simulink model "IEEE33BusTestSystem_DG_Ident"  (R2019a)
settings: Solver=VariableStepAuto  StartTime=0.0  StopTime=1.5  FixedStep=5e-5  RelTol=1e-3
values from neighbouring files (symbols this model uses):
  P_dg0 = 300*ones(1,6)    [IEEE33BusSystem_Control_Sim.m]    (also in IEEE33BusSystem_Control_Sim_nq3.m; IEEE33BusSystem_Control_Sim_nq5.m; IEEE33BusSystem_Ident.m; IEEE33BusSystem_op.m)
  P_dgf = 100*ones(1,6)    [IEEE33BusSystem_Control_Sim.m]    (also in IEEE33BusSystem_Control_Sim_nq3.m; IEEE33BusSystem_Control_Sim_nq5.m; IEEE33BusSystem_op.m = 300*ones(1,6); Kimc_d1_sce1-0.mat = [100 100 100 100 100 100])
  Q_dg0 = zeros(1,6)    [IEEE33BusSystem_Control_Sim.m]    (also in IEEE33BusSystem_Control_Sim_nq3.m; IEEE33BusSystem_Control_Sim_nq5.m; IEEE33BusSystem_Ident.m; IEEE33BusSystem_op.m)
  Q_dgf = zeros(1,6)    [IEEE33BusSystem_op.m]
  Tp = 500e-3    (= 0.5)    [IEEE33BusSystem.m]    (also in Kimc_d1_sce1-0.mat = 0.05; Kimc_d1_sce1-1.mat = 0.05; Kimc_d1_sce1-2.mat = 0.05; Kimc_d1_sce1-3.mat = 0.05)
  tPdg = 10*ones(1,6)    [IEEE33BusSystem_Control_Sim.m]    (also in IEEE33BusSystem_Control_Sim_nq3.m; IEEE33BusSystem_Control_Sim_nq5.m; IEEE33BusSystem_op.m = 0.5*ones(1,6); Kimc_d1_sce1-0.mat = [10 10 10 10 10 10])
  Tq = 50e-3    (= 0.05)    [IEEE33BusSystem.m]    (also in Kimc_d1_sce1-0.mat; Kimc_d1_sce1-1.mat; Kimc_d1_sce1-2.mat; Kimc_d1_sce1-3.mat)
  tQdg = 0.5*ones(1,6)    [IEEE33BusSystem_op.m]
  v0 = ones(1,33)    [IEEE33BusSystem_Control_Sim.m]    (also in IEEE33BusSystem_Control_Sim_nq3.m; IEEE33BusSystem_Control_Sim_nq5.m; IEEE33BusSystem_Ident.m; IEEE33BusSystem_op.m)
  V_0 = v0_sim(CVs_sel)    [IEEE33BusSystem_Control_Sim.m]    (also in IEEE33BusSystem_Control_Sim_nq3.m = [v0_sim(14), v0_sim(18), v0_sim(21), v0_sim(25), v0_sim(30),; IEEE33BusSystem_Control_Sim_nq5.m = [v0_sim(14), v0_sim(18), v0_sim(21), v0_sim(25), v0_sim(30),; IEEE33BusSystem_Ident.m; IEEE33BusSystem_op.m = [v0(14), v0(18), v0(21), v0(25), v0(30), v0(33)])
libraries: powerlib x159, powerlib_meascontrol x33
(part 3 of 3)

== system IEEE33BusTestSystem_DG_Ident/Bus_32 ==
  Bus Load 32 : powerlib/Elements/Three-Phase Series RLC Load  LConnTagsString=A|B|C  Configuration=Y (grounded)  NominalVoltage=(12660)*v0(32)  Vabc=[1e3 1e3 1e3]  Vabcp=[1e3 1e3 1e3]  NominalFrequency=50  UnbalancedPower=off  ActivePower=210e3  InductivePower=100e3  CapacitivePower=0  Pabc=[10e3 9e3 11e3]  QLabc=[100 90 110]  QCabc=[100 90 110]  Pabcp=[10e3 9e3 11e3]  QLabcp=[100 90 110]  QCabcp=[100 90 110]  Measurements=None  LoadType=constant PQ
      settings: SourceProductName=Simscape Electrical
  Bus_32 : powerlib/Measurements/Three-Phase V-I Measurement  VoltageMeasurement=phase-to-phase  SetLabelV=on  LabelV=v32_pu  Vpu=off  VpuLL=on  CurrentMeasurement=yes  SetLabelI=on  LabelI=I3132_pu  Ipu=off  Pbase=100e6  Vbase=12660  OutputType=Complex  PhasorSimulation=on  PSBequivalent=0
      settings: SourceProductName=Simscape Electrical
  CB3-2 : powerlib/Elements/Three-Phase Breaker  InitialState=open  SwitchA=on  SwitchB=on  SwitchC=on  SwitchTimes="[1/60  5/60]"  External=on  BreakerResistance=0.01  SnubberResistance=1e6  SnubberCapacitance=inf  Measurements=None
      settings: SourceProductName=Simscape Electrical
  InPhaseA : PMIOPort  Side=Left
  InPhaseB : PMIOPort  Port=2  Side=Left
  InPhaseC : PMIOPort  Port=3  Side=Left
  OutPhaseA : PMIOPort  Port=4  Side=Right
  OutPhaseB : PMIOPort  Port=5  Side=Right
  OutPhaseC : PMIOPort  Port=6  Side=Right
  wires:
  [CB32to33] -> CB3-2/1
  connections:
  Bus_32/RConn1 -- CB3-2/LConn1 -- Bus Load 32/LConn1
  CB3-2/RConn3 -- OutPhaseC/RConn1
  Bus Load 32/LConn2 -- CB3-2/LConn2 -- Bus_32/RConn2
  Bus_32/RConn3 -- Bus Load 32/LConn3 -- CB3-2/LConn3
  CB3-2/RConn1 -- OutPhaseA/RConn1
  CB3-2/RConn2 -- OutPhaseB/RConn1
  InPhaseA/RConn1 -- Bus_32/LConn1
  InPhaseB/RConn1 -- Bus_32/LConn2
  InPhaseC/RConn1 -- Bus_32/LConn3

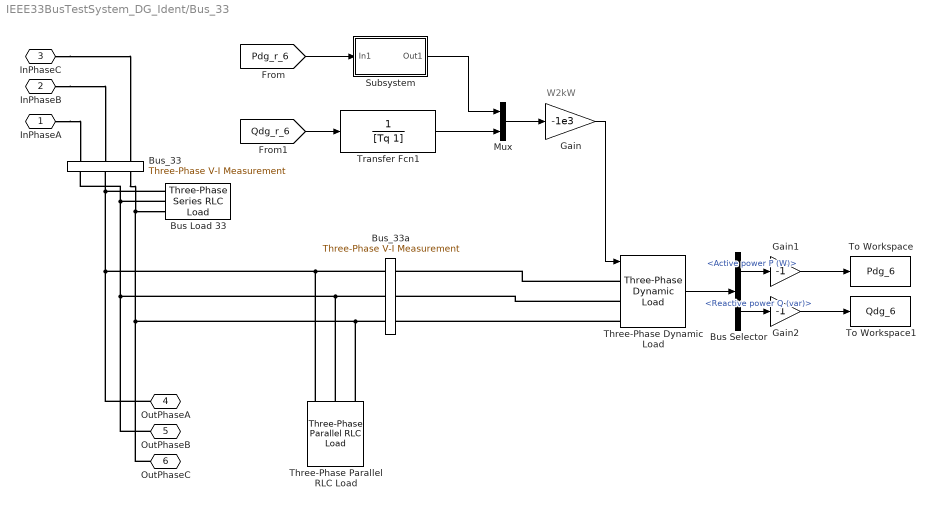
== system IEEE33BusTestSystem_DG_Ident/Bus_33 ==
  note: W2kW
  Bus Load 33 : powerlib/Elements/Three-Phase Series RLC Load  LConnTagsString=A|B|C  Configuration=Y (grounded)  NominalVoltage=(12660)*v0(33)  Vabc=[1e3 1e3 1e3]  Vabcp=[1e3 1e3 1e3]  NominalFrequency=50  UnbalancedPower=off  ActivePower=60e3  InductivePower=40e3  CapacitivePower=0  Pabc=[10e3 9e3 11e3]  QLabc=[100 90 110]  QCabc=[100 90 110]  Pabcp=[10e3 9e3 11e3]  QLabcp=[100 90 110]  QCabcp=[100 90 110]  Measurements=None  LoadType=constant PQ
      settings: SourceProductName=Simscape Electrical
  Bus Selector : BusSelector  OutputSignals=Active power P (W),Reactive power Q (var)
  Bus_33 : powerlib/Measurements/Three-Phase V-I Measurement  VoltageMeasurement=phase-to-phase  SetLabelV=on  LabelV=v33_pu  Vpu=off  VpuLL=on  CurrentMeasurement=yes  SetLabelI=on  LabelI=Iabc  Ipu=off  Pbase=100e6  Vbase=12660  OutputType=Complex  PhasorSimulation=on  PSBequivalent=0
      settings: SourceProductName=Simscape Electrical
  Bus_33a : powerlib/Measurements/Three-Phase V-I Measurement  VoltageMeasurement=no  SetLabelV=off  LabelV=v14a_pu  Vpu=off  VpuLL=off  CurrentMeasurement=yes  SetLabelI=on  LabelI=I33a_pu  Ipu=off  Pbase=100e6  Vbase=500e3  OutputType=Complex  PhasorSimulation=on  PSBequivalent=0
      settings: SourceProductName=Simscape Electrical
  Gain : Gain  Gain=-1e3
  Gain1 : Gain  Gain=-1
  Gain2 : Gain  Gain=-1
  Mux : Mux  Inputs=2
  Subsystem : Subsystem
  Three-Phase Dynamic Load : powerlib/Elements/Three-Phase Dynamic Load  NominalVoltage=[ 12660 50 ]  ActiveReactivePowers=[-P_dg0(6) Q_dg0(6)]*1e3  PositiveSequence=[V_0(6) 0]  ExternalControl=on  NpNq=[1.3 2]  TimeConstants="[0  0  0  0]"  MinimumVoltage=0.7  Tfilter=1e-4  LoadFlowParameters=[4,0,0,0,0]
      settings: SourceProductName=Simscape Electrical  SourceProductBaseCode=PS
  Three-Phase Parallel RLC Load : powerlib/Elements/Three-Phase Parallel RLC Load  LConnTagsString=A|B|C  Configuration=Y (grounded)  NominalVoltage=12660  Vabc=[1e3 1e3 1e3]  Vabcp=[1e3 1e3 1e3]  NominalFrequency=50  UnbalancedPower=off  ActivePower=0.01  InductivePower=0  CapacitivePower=0  Pabc=[10e3 9e3 11e3]  QLabc=[100 90 110]  QCabc=[100 90 110]  Pabcp=[10e3 9e3 11e3]  QLabcp=[100 90 110]  QCabcp=[100 90 110]  Measurements=None  LoadType=constant Z
      settings: SourceProductName=Simscape Electrical
  To Workspace : ToWorkspace  VariableName=Pdg_6  SaveFormat=Timeseries  SampleTime=-1
  To Workspace1 : ToWorkspace  VariableName=Qdg_6  SaveFormat=Timeseries  SampleTime=-1
  Transfer Fcn1 : TransferFcn  Denominator=[Tq 1]
  InPhaseA : PMIOPort  Side=Left
  InPhaseB : PMIOPort  Port=2  Side=Left
  InPhaseC : PMIOPort  Port=3  Side=Left
  OutPhaseA : PMIOPort  Port=4  Side=Right
  OutPhaseB : PMIOPort  Port=5  Side=Right
  OutPhaseC : PMIOPort  Port=6  Side=Right
  wires:
  Subsystem/1(Out1) -> Mux/1
  Transfer Fcn1/1 -> Mux/2
  Bus Selector/1 -> Gain1/1  "<Active power P (W)>"
  [Pdg_r_6] -> Subsystem/1(In1)
  Gain2/1 -> To Workspace1/1
  Bus Selector/2 -> Gain2/1  "<Reactive power Q (var)>"
  Mux/1 -> Gain/1
  Three-Phase Dynamic Load/1 -> Bus Selector/1
  Gain/1 -> Three-Phase Dynamic Load/1
  Gain1/1 -> To Workspace/1
  [Qdg_r_6] -> Transfer Fcn1/1
  connections:
  Bus Load 33/LConn1 -- Three-Phase Parallel RLC Load/LConn1 -- Bus_33a/RConn1 -- OutPhaseA/RConn1 -- Bus_33/RConn1
  Bus Load 33/LConn2 -- Three-Phase Parallel RLC Load/LConn2 -- Bus_33a/RConn2 -- OutPhaseB/RConn1 -- Bus_33/RConn2
  Bus_33/RConn3 -- Three-Phase Parallel RLC Load/LConn3 -- Bus_33a/RConn3 -- OutPhaseC/RConn1 -- Bus Load 33/LConn3
  InPhaseA/RConn1 -- Bus_33/LConn1
  InPhaseB/RConn1 -- Bus_33/LConn2
  InPhaseC/RConn1 -- Bus_33/LConn3
  Three-Phase Dynamic Load/LConn1 -- Bus_33a/LConn1
  Three-Phase Dynamic Load/LConn3 -- Bus_33a/LConn3
  Three-Phase Dynamic Load/LConn2 -- Bus_33a/LConn2

== system IEEE33BusTestSystem_DG_Ident/Bus_4 ==
  Bus Load 4 : powerlib/Elements/Three-Phase Series RLC Load  LConnTagsString=A|B|C  Configuration=Y (grounded)  NominalVoltage=(12660)*v0(4)  Vabc=[1e3 1e3 1e3]  Vabcp=[1e3 1e3 1e3]  NominalFrequency=50  UnbalancedPower=off  ActivePower=120e3  InductivePower=80e3  CapacitivePower=0  Pabc=[10e3 9e3 11e3]  QLabc=[100 90 110]  QCabc=[100 90 110]  Pabcp=[10e3 9e3 11e3]  QLabcp=[100 90 110]  QCabcp=[100 90 110]  Measurements=None  LoadType=constant PQ
      settings: SourceProductName=Simscape Electrical
  Bus_4 : powerlib/Measurements/Three-Phase V-I Measurement  VoltageMeasurement=phase-to-phase  SetLabelV=on  LabelV=v4_pu  Vpu=off  VpuLL=on  CurrentMeasurement=yes  SetLabelI=on  LabelI=I34_pu  Ipu=off  Pbase=10e6  Vbase=12660  OutputType=Complex  PhasorSimulation=on  PSBequivalent=0
      settings: SourceProductName=Simscape Electrical
  CB3-2 : powerlib/Elements/Three-Phase Breaker  InitialState=open  SwitchA=on  SwitchB=on  SwitchC=on  SwitchTimes="[1/60  5/60]"  External=on  BreakerResistance=0.01  SnubberResistance=1e6  SnubberCapacitance=inf  Measurements=None
      settings: SourceProductName=Simscape Electrical
  InPhaseA : PMIOPort  Side=Left
  InPhaseB : PMIOPort  Port=2  Side=Left
  InPhaseC : PMIOPort  Port=3  Side=Left
  OutPhaseA : PMIOPort  Port=4  Side=Right
  OutPhaseB : PMIOPort  Port=5  Side=Right
  OutPhaseC : PMIOPort  Port=6  Side=Right
  wires:
  [CB4to5] -> CB3-2/1
  connections:
  Bus_4/RConn1 -- CB3-2/LConn1 -- Bus Load 4/LConn1
  CB3-2/RConn3 -- OutPhaseC/RConn1
  Bus Load 4/LConn2 -- CB3-2/LConn2 -- Bus_4/RConn2
  Bus_4/RConn3 -- CB3-2/LConn3 -- Bus Load 4/LConn3
  CB3-2/RConn1 -- OutPhaseA/RConn1
  CB3-2/RConn2 -- OutPhaseB/RConn1
  InPhaseA/RConn1 -- Bus_4/LConn1
  InPhaseB/RConn1 -- Bus_4/LConn2
  InPhaseC/RConn1 -- Bus_4/LConn3

== system IEEE33BusTestSystem_DG_Ident/Bus_5 ==
  Bus Load 5 : powerlib/Elements/Three-Phase Series RLC Load  LConnTagsString=A|B|C  Configuration=Y (grounded)  NominalVoltage=(12660)*v0(5)  Vabc=[1e3 1e3 1e3]  Vabcp=[1e3 1e3 1e3]  NominalFrequency=50  UnbalancedPower=off  ActivePower=60e3  InductivePower=30e3  CapacitivePower=0  Pabc=[10e3 9e3 11e3]  QLabc=[100 90 110]  QCabc=[100 90 110]  Pabcp=[10e3 9e3 11e3]  QLabcp=[100 90 110]  QCabcp=[100 90 110]  Measurements=None  LoadType=constant PQ
      settings: SourceProductName=Simscape Electrical
  Bus_5 : powerlib/Measurements/Three-Phase V-I Measurement  VoltageMeasurement=phase-to-phase  SetLabelV=on  LabelV=v5_pu  Vpu=off  VpuLL=on  CurrentMeasurement=yes  SetLabelI=on  LabelI=I45_pu  Ipu=off  Pbase=10e6  Vbase=12660  OutputType=Complex  PhasorSimulation=on  PSBequivalent=0
      settings: SourceProductName=Simscape Electrical
  CB3-2 : powerlib/Elements/Three-Phase Breaker  InitialState=open  SwitchA=on  SwitchB=on  SwitchC=on  SwitchTimes="[1/60  5/60]"  External=on  BreakerResistance=0.01  SnubberResistance=1e6  SnubberCapacitance=inf  Measurements=None
      settings: SourceProductName=Simscape Electrical
  InPhaseA : PMIOPort  Side=Left
  InPhaseB : PMIOPort  Port=2  Side=Left
  InPhaseC : PMIOPort  Port=3  Side=Left
  OutPhaseA : PMIOPort  Port=4  Side=Right
  OutPhaseB : PMIOPort  Port=5  Side=Right
  OutPhaseC : PMIOPort  Port=6  Side=Right
  wires:
  [CB5to6] -> CB3-2/1
  connections:
  Bus Load 5/LConn1 -- CB3-2/LConn1 -- Bus_5/RConn1
  CB3-2/RConn3 -- OutPhaseC/RConn1
  Bus_5/RConn2 -- CB3-2/LConn2 -- Bus Load 5/LConn2
  Bus_5/RConn3 -- CB3-2/LConn3 -- Bus Load 5/LConn3
  CB3-2/RConn1 -- OutPhaseA/RConn1
  CB3-2/RConn2 -- OutPhaseB/RConn1
  InPhaseA/RConn1 -- Bus_5/LConn1
  InPhaseB/RConn1 -- Bus_5/LConn2
  InPhaseC/RConn1 -- Bus_5/LConn3

== system IEEE33BusTestSystem_DG_Ident/Bus_6 ==
  Bus Load 6 : powerlib/Elements/Three-Phase Series RLC Load  LConnTagsString=A|B|C  Configuration=Y (grounded)  NominalVoltage=(12660)*v0(6)  Vabc=[1e3 1e3 1e3]  Vabcp=[1e3 1e3 1e3]  NominalFrequency=50  UnbalancedPower=off  ActivePower=60e3  InductivePower=20e3  CapacitivePower=0  Pabc=[10e3 9e3 11e3]  QLabc=[100 90 110]  QCabc=[100 90 110]  Pabcp=[10e3 9e3 11e3]  QLabcp=[100 90 110]  QCabcp=[100 90 110]  Measurements=None  LoadType=constant PQ
      settings: SourceProductName=Simscape Electrical
  Bus_6 : powerlib/Measurements/Three-Phase V-I Measurement  VoltageMeasurement=phase-to-phase  SetLabelV=on  LabelV=v6_pu  Vpu=off  VpuLL=on  CurrentMeasurement=yes  SetLabelI=on  LabelI=I56_pu  Ipu=off  Pbase=100e6  Vbase=12660  OutputType=Complex  PhasorSimulation=on  PSBequivalent=0
      settings: SourceProductName=Simscape Electrical
  CB3-1 : powerlib/Elements/Three-Phase Breaker  InitialState=open  SwitchA=on  SwitchB=on  SwitchC=on  SwitchTimes="[1/60  5/60]"  External=on  BreakerResistance=0.01  SnubberResistance=1e6  SnubberCapacitance=inf  Measurements=None
      settings: SourceProductName=Simscape Electrical
  CB3-2 : powerlib/Elements/Three-Phase Breaker  InitialState=open  SwitchA=on  SwitchB=on  SwitchC=on  SwitchTimes="[1/60  5/60]"  External=on  BreakerResistance=0.01  SnubberResistance=1e6  SnubberCapacitance=inf  Measurements=None
      settings: SourceProductName=Simscape Electrical
  InPhaseA : PMIOPort  Side=Left
  InPhaseB : PMIOPort  Port=2  Side=Left
  InPhaseC : PMIOPort  Port=3  Side=Left
  OutPhaseA : PMIOPort  Port=4  Side=Right
  OutPhaseB : PMIOPort  Port=5  Side=Right
  OutPhaseC : PMIOPort  Port=6  Side=Right
  OutPhaseA1 : PMIOPort  Port=7  Side=Right
  OutPhaseB1 : PMIOPort  Port=8  Side=Right
  OutPhaseC1 : PMIOPort  Port=9  Side=Right
  wires:
  [CB6to26] -> CB3-1/1
  [CB6to7] -> CB3-2/1
  connections:
  Bus Load 6/LConn1 -- Bus_6/RConn1 -- CB3-2/LConn1 -- CB3-1/LConn1
  CB3-2/RConn3 -- OutPhaseC/RConn1
  Bus Load 6/LConn2 -- Bus_6/RConn2 -- CB3-1/LConn2 -- CB3-2/LConn2
  Bus Load 6/LConn3 -- Bus_6/RConn3 -- CB3-1/LConn3 -- CB3-2/LConn3
  CB3-2/RConn1 -- OutPhaseA/RConn1
  CB3-2/RConn2 -- OutPhaseB/RConn1
  CB3-1/RConn3 -- OutPhaseC1/RConn1
  CB3-1/RConn2 -- OutPhaseB1/RConn1
  CB3-1/RConn1 -- OutPhaseA1/RConn1
  InPhaseA/RConn1 -- Bus_6/LConn1
  InPhaseB/RConn1 -- Bus_6/LConn2
  InPhaseC/RConn1 -- Bus_6/LConn3

== system IEEE33BusTestSystem_DG_Ident/Bus_7 ==
  Bus Load 7 : powerlib/Elements/Three-Phase Series RLC Load  LConnTagsString=A|B|C  Configuration=Y (grounded)  NominalVoltage=(12660)*v0(7)  Vabc=[1e3 1e3 1e3]  Vabcp=[1e3 1e3 1e3]  NominalFrequency=50  UnbalancedPower=off  ActivePower=200e3  InductivePower=100e3  CapacitivePower=0  Pabc=[10e3 9e3 11e3]  QLabc=[100 90 110]  QCabc=[100 90 110]  Pabcp=[10e3 9e3 11e3]  QLabcp=[100 90 110]  QCabcp=[100 90 110]  Measurements=None  LoadType=constant PQ
      settings: SourceProductName=Simscape Electrical
  Bus_7 : powerlib/Measurements/Three-Phase V-I Measurement  VoltageMeasurement=phase-to-phase  SetLabelV=on  LabelV=v7_pu  Vpu=off  VpuLL=on  CurrentMeasurement=yes  SetLabelI=on  LabelI=I67_pu  Ipu=off  Pbase=100e6  Vbase=12660  OutputType=Complex  PhasorSimulation=on  PSBequivalent=0
      settings: SourceProductName=Simscape Electrical
  CB3-2 : powerlib/Elements/Three-Phase Breaker  InitialState=open  SwitchA=on  SwitchB=on  SwitchC=on  SwitchTimes="[1/60  5/60]"  External=on  BreakerResistance=0.01  SnubberResistance=1e6  SnubberCapacitance=inf  Measurements=None
      settings: SourceProductName=Simscape Electrical
  InPhaseA : PMIOPort  Side=Left
  InPhaseB : PMIOPort  Port=2  Side=Left
  InPhaseC : PMIOPort  Port=3  Side=Left
  OutPhaseA : PMIOPort  Port=4  Side=Right
  OutPhaseB : PMIOPort  Port=5  Side=Right
  OutPhaseC : PMIOPort  Port=6  Side=Right
  wires:
  [CB7to8] -> CB3-2/1
  connections:
  Bus_7/RConn1 -- CB3-2/LConn1 -- Bus Load 7/LConn1
  CB3-2/RConn3 -- OutPhaseC/RConn1
  Bus Load 7/LConn2 -- CB3-2/LConn2 -- Bus_7/RConn2
  CB3-2/LConn3 -- Bus Load 7/LConn3 -- Bus_7/RConn3
  CB3-2/RConn1 -- OutPhaseA/RConn1
  CB3-2/RConn2 -- OutPhaseB/RConn1
  InPhaseA/RConn1 -- Bus_7/LConn1
  InPhaseB/RConn1 -- Bus_7/LConn2
  InPhaseC/RConn1 -- Bus_7/LConn3

== system IEEE33BusTestSystem_DG_Ident/Bus_8 ==
  Bus Load 8 : powerlib/Elements/Three-Phase Series RLC Load  LConnTagsString=A|B|C  Configuration=Y (grounded)  NominalVoltage=(12660)*v0(8)  Vabc=[1e3 1e3 1e3]  Vabcp=[1e3 1e3 1e3]  NominalFrequency=50  UnbalancedPower=off  ActivePower=200e3  InductivePower=100e3  CapacitivePower=0  Pabc=[10e3 9e3 11e3]  QLabc=[100 90 110]  QCabc=[100 90 110]  Pabcp=[10e3 9e3 11e3]  QLabcp=[100 90 110]  QCabcp=[100 90 110]  Measurements=None  LoadType=constant PQ
      settings: SourceProductName=Simscape Electrical
  Bus_8 : powerlib/Measurements/Three-Phase V-I Measurement  VoltageMeasurement=phase-to-phase  SetLabelV=on  LabelV=v8_pu  Vpu=off  VpuLL=on  CurrentMeasurement=yes  SetLabelI=on  LabelI=I78_pu  Ipu=off  Pbase=100e6  Vbase=12660  OutputType=Complex  PhasorSimulation=on  PSBequivalent=0
      settings: SourceProductName=Simscape Electrical
  CB3-2 : powerlib/Elements/Three-Phase Breaker  InitialState=open  SwitchA=on  SwitchB=on  SwitchC=on  SwitchTimes="[1/60  5/60]"  External=on  BreakerResistance=0.01  SnubberResistance=1e6  SnubberCapacitance=inf  Measurements=None
      settings: SourceProductName=Simscape Electrical
  InPhaseA : PMIOPort  Side=Left
  InPhaseB : PMIOPort  Port=2  Side=Left
  InPhaseC : PMIOPort  Port=3  Side=Left
  OutPhaseA : PMIOPort  Port=4  Side=Right
  OutPhaseB : PMIOPort  Port=5  Side=Right
  OutPhaseC : PMIOPort  Port=6  Side=Right
  InPhaseA1 : PMIOPort  Port=7  Side=Left
  InPhaseB1 : PMIOPort  Port=8  Side=Left
  InPhaseC1 : PMIOPort  Port=9  Side=Left
  wires:
  [CB8to9] -> CB3-2/1
  connections:
  Bus Load 8/LConn1 -- CB3-2/LConn1 -- Bus_8/RConn1
  CB3-2/RConn3 -- OutPhaseC/RConn1
  Bus Load 8/LConn2 -- CB3-2/LConn2 -- Bus_8/RConn2
  Bus_8/RConn3 -- CB3-2/LConn3 -- Bus Load 8/LConn3
  CB3-2/RConn1 -- OutPhaseA/RConn1
  CB3-2/RConn2 -- OutPhaseB/RConn1
  InPhaseA1/RConn1 -- InPhaseA/RConn1 -- Bus_8/LConn1
  InPhaseB1/RConn1 -- InPhaseB/RConn1 -- Bus_8/LConn2
  InPhaseC1/RConn1 -- InPhaseC/RConn1 -- Bus_8/LConn3

== system IEEE33BusTestSystem_DG_Ident/Bus_9 ==
  Bus Load 9 : powerlib/Elements/Three-Phase Series RLC Load  LConnTagsString=A|B|C  Configuration=Y (grounded)  NominalVoltage=(12660)*v0(9)  Vabc=[1e3 1e3 1e3]  Vabcp=[1e3 1e3 1e3]  NominalFrequency=50  UnbalancedPower=off  ActivePower=60e3  InductivePower=20e3  CapacitivePower=0  Pabc=[10e3 9e3 11e3]  QLabc=[100 90 110]  QCabc=[100 90 110]  Pabcp=[10e3 9e3 11e3]  QLabcp=[100 90 110]  QCabcp=[100 90 110]  Measurements=None  LoadType=constant PQ
      settings: SourceProductName=Simscape Electrical
  Bus_9 : powerlib/Measurements/Three-Phase V-I Measurement  VoltageMeasurement=phase-to-phase  SetLabelV=on  LabelV=v9_pu  Vpu=off  VpuLL=on  CurrentMeasurement=yes  SetLabelI=on  LabelI=I89_pu  Ipu=off  Pbase=100e6  Vbase=12660  OutputType=Complex  PhasorSimulation=on  PSBequivalent=0
      settings: SourceProductName=Simscape Electrical
  CB3-1 : powerlib/Elements/Three-Phase Breaker  InitialState=open  SwitchA=on  SwitchB=on  SwitchC=on  SwitchTimes="[1/60  5/60]"  External=on  BreakerResistance=0.01  SnubberResistance=1e6  SnubberCapacitance=inf  Measurements=None
      settings: SourceProductName=Simscape Electrical
  CB3-2 : powerlib/Elements/Three-Phase Breaker  InitialState=open  SwitchA=on  SwitchB=on  SwitchC=on  SwitchTimes="[1/60  5/60]"  External=on  BreakerResistance=0.01  SnubberResistance=1e6  SnubberCapacitance=inf  Measurements=None
      settings: SourceProductName=Simscape Electrical
  InPhaseA : PMIOPort  Side=Left
  InPhaseB : PMIOPort  Port=2  Side=Left
  InPhaseC : PMIOPort  Port=3  Side=Left
  OutPhaseA : PMIOPort  Port=4  Side=Right
  OutPhaseB : PMIOPort  Port=5  Side=Right
  OutPhaseC : PMIOPort  Port=6  Side=Right
  OutPhaseA1 : PMIOPort  Port=7  Side=Right
  OutPhaseB1 : PMIOPort  Port=8  Side=Right
  OutPhaseC1 : PMIOPort  Port=9  Side=Right
  wires:
  [CB9to10] -> CB3-2/1
  [CB9to15] -> CB3-1/1
  connections:
  CB3-1/LConn1 -- Bus Load 9/LConn1 -- Bus_9/RConn1 -- CB3-2/LConn1
  CB3-2/RConn3 -- OutPhaseC/RConn1
  CB3-1/LConn2 -- Bus_9/RConn2 -- Bus Load 9/LConn2 -- CB3-2/LConn2
  Bus Load 9/LConn3 -- Bus_9/RConn3 -- CB3-1/LConn3 -- CB3-2/LConn3
  CB3-2/RConn1 -- OutPhaseA/RConn1
  CB3-2/RConn2 -- OutPhaseB/RConn1
  InPhaseA/RConn1 -- Bus_9/LConn1
  InPhaseB/RConn1 -- Bus_9/LConn2
  InPhaseC/RConn1 -- Bus_9/LConn3
  CB3-1/RConn2 -- OutPhaseB1/RConn1
  CB3-1/RConn3 -- OutPhaseC1/RConn1
  CB3-1/RConn1 -- OutPhaseA1/RConn1

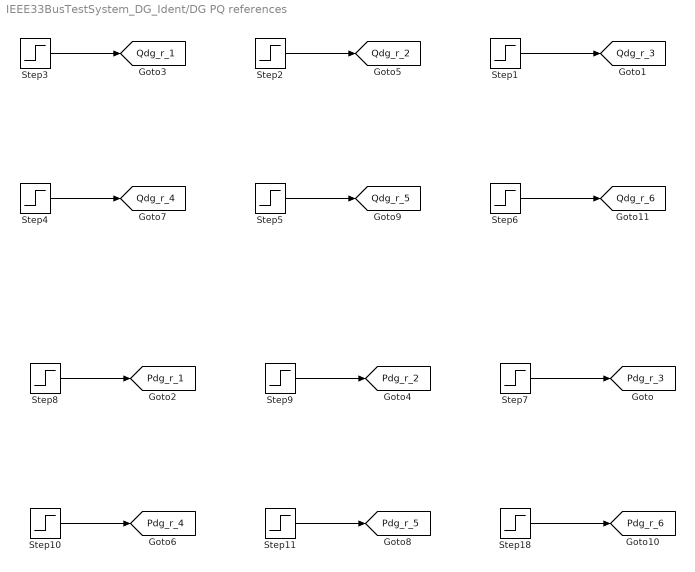
== system IEEE33BusTestSystem_DG_Ident/DG PQ references ==
  Step1 : Step  Time=tQdg(3)  Before=Q_dg0(3)  After=Q_dgf(3)  SampleTime=0
  Step10 : Step  Time=tPdg(4)  Before=P_dg0(4)  After=P_dgf(4)  SampleTime=0
  Step11 : Step  Time=tPdg(5)  Before=P_dg0(5)  After=P_dgf(5)  SampleTime=0
  Step18 : Step  Time=tPdg(6)  Before=P_dg0(6)  After=P_dgf(6)  SampleTime=0
  Step2 : Step  Time=tQdg(2)  Before=Q_dg0(2)  After=Q_dgf(2)  SampleTime=0
  Step3 : Step  Time=tQdg(1)  Before=Q_dg0(1)  After=Q_dgf(1)  SampleTime=0
  Step4 : Step  Time=tQdg(4)  Before=Q_dg0(4)  After=Q_dgf(4)  SampleTime=0
  Step5 : Step  Time=tQdg(5)  Before=Q_dg0(5)  After=Q_dgf(5)  SampleTime=0
  Step6 : Step  Time=tQdg(6)  Before=Q_dg0(6)  After=Q_dgf(6)  SampleTime=0
  Step7 : Step  Time=tPdg(3)  Before=P_dg0(3)  After=P_dgf(3)  SampleTime=0
  Step8 : Step  Time=tPdg(1)  Before=P_dg0(1)  After=P_dgf(1)  SampleTime=0
  Step9 : Step  Time=tPdg(2)  Before=P_dg0(2)  After=P_dgf(2)  SampleTime=0
  tag scope: Pdg_r_1=global, Pdg_r_2=global, Pdg_r_3=global, Pdg_r_4=global, Pdg_r_5=global, Pdg_r_6=global, Qdg_r_1=global, Qdg_r_2=global, Qdg_r_3=global, Qdg_r_4=global, Qdg_r_5=global, Qdg_r_6=global
  wires:
  Step1/1 -> [Qdg_r_3]
  Step3/1 -> [Qdg_r_1]
  Step2/1 -> [Qdg_r_2]
  Step4/1 -> [Qdg_r_4]
  Step5/1 -> [Qdg_r_5]
  Step6/1 -> [Qdg_r_6]
  Step18/1 -> [Pdg_r_6]
  Step10/1 -> [Pdg_r_4]
  Step9/1 -> [Pdg_r_2]
  Step8/1 -> [Pdg_r_1]
  Step7/1 -> [Pdg_r_3]
  Step11/1 -> [Pdg_r_5]

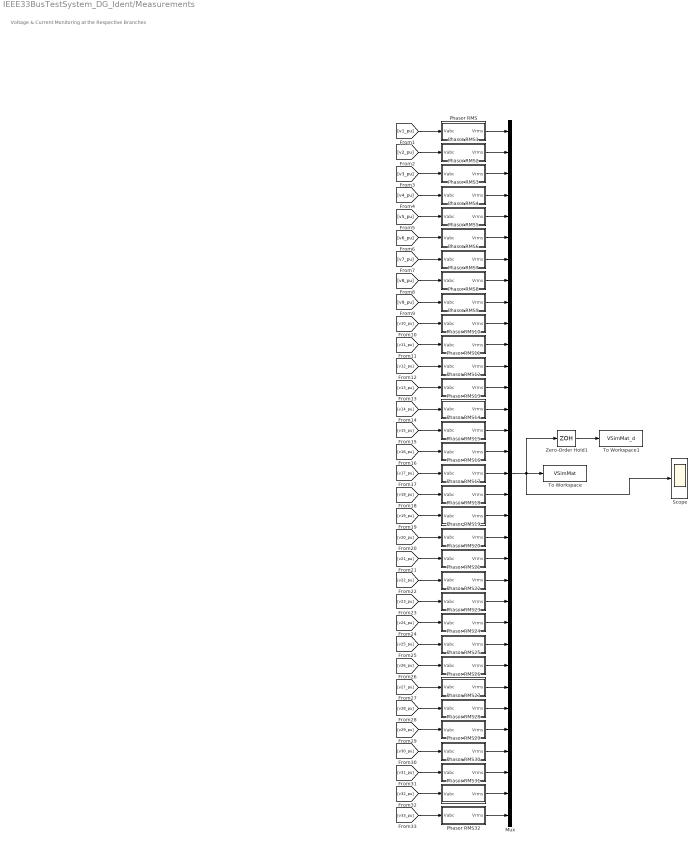
== system IEEE33BusTestSystem_DG_Ident/Measurements ==
  note: Voltage & Current Monitoring at the Respective Branches
  Mux : Mux  Inputs=33
  Phasor RMS : Subsystem
  Phasor RMS1 : Subsystem
  Phasor RMS10 : Subsystem
  Phasor RMS11 : Subsystem
  Phasor RMS12 : Subsystem
  Phasor RMS13 : Subsystem
  Phasor RMS14 : Subsystem
  Phasor RMS15 : Subsystem
  Phasor RMS16 : Subsystem
  Phasor RMS17 : Subsystem
  Phasor RMS18 : Subsystem
  Phasor RMS19 : Subsystem
  Phasor RMS2 : Subsystem
  Phasor RMS20 : Subsystem
  Phasor RMS21 : Subsystem
  Phasor RMS22 : Subsystem
  Phasor RMS23 : Subsystem
  Phasor RMS24 : Subsystem
  Phasor RMS25 : Subsystem
  Phasor RMS26 : Subsystem
  Phasor RMS27 : Subsystem
  Phasor RMS28 : Subsystem
  Phasor RMS29 : Subsystem
  Phasor RMS3 : Subsystem
  Phasor RMS30 : Subsystem
  Phasor RMS31 : Subsystem
  Phasor RMS32 : Subsystem
  Phasor RMS4 : Subsystem
  Phasor RMS5 : Subsystem
  Phasor RMS6 : Subsystem
  Phasor RMS7 : Subsystem
  Phasor RMS8 : Subsystem
  Phasor RMS9 : Subsystem
  Scope : Scope
  To Workspace : ToWorkspace  VariableName=VSimMat  SampleTime=-1
  To Workspace1 : ToWorkspace  VariableName=VSimMat_d  SampleTime=-1
  Zero-Order Hold1 : ZeroOrderHold  SampleTime=0.005
  wires:
  [v33_pu] -> Phasor RMS32/1(Vabc)
  [v15_pu] -> Phasor RMS14/1(Vabc)
  [v4_pu] -> Phasor RMS3/1(Vabc)
  [v23_pu] -> Phasor RMS22/1(Vabc)
  Phasor RMS4/1(Vrms) -> Mux/5
  Phasor RMS11/1(Vrms) -> Mux/12
  [v32_pu] -> Phasor RMS31/1(Vabc)
  Phasor RMS/1(Vrms) -> Mux/1
  Phasor RMS3/1(Vrms) -> Mux/4
  Phasor RMS30/1(Vrms) -> Mux/31
  Phasor RMS26/1(Vrms) -> Mux/27
  [v25_pu] -> Phasor RMS24/1(Vabc)
  Phasor RMS27/1(Vrms) -> Mux/28
  Phasor RMS28/1(Vrms) -> Mux/29
  Phasor RMS17/1(Vrms) -> Mux/18
  Phasor RMS9/1(Vrms) -> Mux/10
  [v20_pu] -> Phasor RMS19/1(Vabc)
  [v9_pu] -> Phasor RMS8/1(Vabc)
  Phasor RMS5/1(Vrms) -> Mux/6
  [v16_pu] -> Phasor RMS15/1(Vabc)
  Phasor RMS31/1(Vrms) -> Mux/32
  Phasor RMS20/1(Vrms) -> Mux/21
  Phasor RMS6/1(Vrms) -> Mux/7
  Phasor RMS7/1(Vrms) -> Mux/8
  [v30_pu] -> Phasor RMS29/1(Vabc)
  [v2_pu] -> Phasor RMS1/1(Vabc)
  Phasor RMS19/1(Vrms) -> Mux/20
  [v17_pu] -> Phasor RMS16/1(Vabc)
  Phasor RMS16/1(Vrms) -> Mux/17
  [v13_pu] -> Phasor RMS12/1(Vabc)
  [v14_pu] -> Phasor RMS13/1(Vabc)
  Phasor RMS10/1(Vrms) -> Mux/11
  Phasor RMS22/1(Vrms) -> Mux/23
  [v24_pu] -> Phasor RMS23/1(Vabc)
  Phasor RMS29/1(Vrms) -> Mux/30
  Phasor RMS12/1(Vrms) -> Mux/13
  [v3_pu] -> Phasor RMS2/1(Vabc)
  [v18_pu] -> Phasor RMS17/1(Vabc)
  [v1_pu] -> Phasor RMS/1(Vabc)
  [v5_pu] -> Phasor RMS4/1(Vabc)
  [v11_pu] -> Phasor RMS10/1(Vabc)
  [v7_pu] -> Phasor RMS6/1(Vabc)
  Phasor RMS2/1(Vrms) -> Mux/3
  [v8_pu] -> Phasor RMS7/1(Vabc)
  [v27_pu] -> Phasor RMS26/1(Vabc)
  Phasor RMS14/1(Vrms) -> Mux/15
  Phasor RMS21/1(Vrms) -> Mux/22
  [v10_pu] -> Phasor RMS9/1(Vabc)
  [v22_pu] -> Phasor RMS21/1(Vabc)
  [v26_pu] -> Phasor RMS25/1(Vabc)
  Phasor RMS1/1(Vrms) -> Mux/2
  Phasor RMS23/1(Vrms) -> Mux/24
  Phasor RMS8/1(Vrms) -> Mux/9
  [v29_pu] -> Phasor RMS28/1(Vabc)
  Phasor RMS25/1(Vrms) -> Mux/26
  [v6_pu] -> Phasor RMS5/1(Vabc)
  Phasor RMS15/1(Vrms) -> Mux/16
  [v12_pu] -> Phasor RMS11/1(Vabc)
  Phasor RMS13/1(Vrms) -> Mux/14
  [v19_pu] -> Phasor RMS18/1(Vabc)
  Phasor RMS18/1(Vrms) -> Mux/19
  [v21_pu] -> Phasor RMS20/1(Vabc)
  [v31_pu] -> Phasor RMS30/1(Vabc)
  [v28_pu] -> Phasor RMS27/1(Vabc)
  Phasor RMS32/1(Vrms) -> Mux/33
  Phasor RMS24/1(Vrms) -> Mux/25
  Zero-Order Hold1/1 -> To Workspace1/1
  Mux/1 -> Zero-Order Hold1/1, To Workspace/1, Scope/1

== system IEEE33BusTestSystem_DG_Ident/Bus_14/Subsystem ==
  In1 : Inport
  Gain : Gain  Gain=1/Tp
  Integrator : Integrator  InitialCondition=P_dg0(1)
  Sum : Sum  Inputs=|+-
  Out1 : Outport
  wires:
  In1/1 -> Sum/1
  Sum/1 -> Gain/1
  Integrator/1 -> Sum/2, Out1/1
  Gain/1 -> Integrator/1

== system IEEE33BusTestSystem_DG_Ident/Bus_18/Subsystem ==
  In1 : Inport
  Gain : Gain  Gain=1/Tp
  Integrator : Integrator  InitialCondition=P_dg0(2)
  Sum : Sum  Inputs=|+-
  Out1 : Outport
  wires:
  In1/1 -> Sum/1
  Sum/1 -> Gain/1
  Integrator/1 -> Sum/2, Out1/1
  Gain/1 -> Integrator/1

== system IEEE33BusTestSystem_DG_Ident/Bus_21/Subsystem ==
  In1 : Inport
  Gain : Gain  Gain=1/Tp
  Integrator : Integrator  InitialCondition=P_dg0(3)
  Sum : Sum  Inputs=|+-
  Out1 : Outport
  wires:
  In1/1 -> Sum/1
  Sum/1 -> Gain/1
  Integrator/1 -> Sum/2, Out1/1
  Gain/1 -> Integrator/1

== system IEEE33BusTestSystem_DG_Ident/Bus_25/Subsystem ==
  In1 : Inport
  Gain : Gain  Gain=1/Tp
  Integrator : Integrator  InitialCondition=P_dg0(4)
  Sum : Sum  Inputs=|+-
  Out1 : Outport
  wires:
  In1/1 -> Sum/1
  Sum/1 -> Gain/1
  Integrator/1 -> Sum/2, Out1/1
  Gain/1 -> Integrator/1

== system IEEE33BusTestSystem_DG_Ident/Bus_30/Subsystem ==
  In1 : Inport
  Gain : Gain  Gain=1/Tp
  Integrator : Integrator  InitialCondition=P_dg0(5)
  Sum : Sum  Inputs=|+-
  Out1 : Outport
  wires:
  In1/1 -> Sum/1
  Sum/1 -> Gain/1
  Integrator/1 -> Sum/2, Out1/1
  Gain/1 -> Integrator/1

== system IEEE33BusTestSystem_DG_Ident/Bus_33/Subsystem ==
  In1 : Inport
  Gain : Gain  Gain=1/Tp
  Integrator : Integrator  InitialCondition=P_dg0(6)
  Sum : Sum  Inputs=|+-
  Out1 : Outport
  wires:
  In1/1 -> Sum/1
  Sum/1 -> Gain/1
  Integrator/1 -> Sum/2, Out1/1
  Gain/1 -> Integrator/1

== system IEEE33BusTestSystem_DG_Ident/Measurements/Phasor RMS ==
  Vabc : Inport
  Sequence Analyzer (Phasor) : powerlib_meascontrol/Measurements/Sequence Analyzer (Phasor)  seq=Positive
      settings: SourceProductName=Simscape Power Systems  SourceProductBaseCode=PS
  Terminator : Terminator
  Vrms : Outport
  wires:
  Sequence Analyzer (Phasor)/1 -> Vrms/1
  Vabc/1 -> Sequence Analyzer (Phasor)/1
  Sequence Analyzer (Phasor)/2 -> Terminator/1

== system IEEE33BusTestSystem_DG_Ident/Measurements/Phasor RMS1 ==
  Vabc : Inport
  Sequence Analyzer (Phasor) : powerlib_meascontrol/Measurements/Sequence Analyzer (Phasor)  seq=Positive
      settings: SourceProductName=Simscape Power Systems  SourceProductBaseCode=PS
  Terminator : Terminator
  Vrms : Outport
  wires:
  Sequence Analyzer (Phasor)/1 -> Vrms/1
  Vabc/1 -> Sequence Analyzer (Phasor)/1
  Sequence Analyzer (Phasor)/2 -> Terminator/1

== system IEEE33BusTestSystem_DG_Ident/Measurements/Phasor RMS10 ==
  Vabc : Inport
  Sequence Analyzer (Phasor) : powerlib_meascontrol/Measurements/Sequence Analyzer (Phasor)  seq=Positive
      settings: SourceProductName=Simscape Power Systems  SourceProductBaseCode=PS
  Terminator : Terminator
  Vrms : Outport
  wires:
  Sequence Analyzer (Phasor)/1 -> Vrms/1
  Vabc/1 -> Sequence Analyzer (Phasor)/1
  Sequence Analyzer (Phasor)/2 -> Terminator/1

== system IEEE33BusTestSystem_DG_Ident/Measurements/Phasor RMS11 ==
  Vabc : Inport
  Sequence Analyzer (Phasor) : powerlib_meascontrol/Measurements/Sequence Analyzer (Phasor)  seq=Positive
      settings: SourceProductName=Simscape Power Systems  SourceProductBaseCode=PS
  Terminator : Terminator
  Vrms : Outport
  wires:
  Sequence Analyzer (Phasor)/1 -> Vrms/1
  Vabc/1 -> Sequence Analyzer (Phasor)/1
  Sequence Analyzer (Phasor)/2 -> Terminator/1

== system IEEE33BusTestSystem_DG_Ident/Measurements/Phasor RMS12 ==
  Vabc : Inport
  Sequence Analyzer (Phasor) : powerlib_meascontrol/Measurements/Sequence Analyzer (Phasor)  seq=Positive
      settings: SourceProductName=Simscape Power Systems  SourceProductBaseCode=PS
  Terminator : Terminator
  Vrms : Outport
  wires:
  Sequence Analyzer (Phasor)/1 -> Vrms/1
  Vabc/1 -> Sequence Analyzer (Phasor)/1
  Sequence Analyzer (Phasor)/2 -> Terminator/1

== system IEEE33BusTestSystem_DG_Ident/Measurements/Phasor RMS13 ==
  Vabc : Inport
  Sequence Analyzer (Phasor) : powerlib_meascontrol/Measurements/Sequence Analyzer (Phasor)  seq=Positive
      settings: SourceProductName=Simscape Power Systems  SourceProductBaseCode=PS
  Terminator : Terminator
  Vrms : Outport
  wires:
  Sequence Analyzer (Phasor)/1 -> Vrms/1
  Vabc/1 -> Sequence Analyzer (Phasor)/1
  Sequence Analyzer (Phasor)/2 -> Terminator/1

== system IEEE33BusTestSystem_DG_Ident/Measurements/Phasor RMS14 ==
  Vabc : Inport
  Sequence Analyzer (Phasor) : powerlib_meascontrol/Measurements/Sequence Analyzer (Phasor)  seq=Positive
      settings: SourceProductName=Simscape Power Systems  SourceProductBaseCode=PS
  Terminator : Terminator
  Vrms : Outport
  wires:
  Sequence Analyzer (Phasor)/1 -> Vrms/1
  Vabc/1 -> Sequence Analyzer (Phasor)/1
  Sequence Analyzer (Phasor)/2 -> Terminator/1

== system IEEE33BusTestSystem_DG_Ident/Measurements/Phasor RMS15 ==
  Vabc : Inport
  Sequence Analyzer (Phasor) : powerlib_meascontrol/Measurements/Sequence Analyzer (Phasor)  seq=Positive
      settings: SourceProductName=Simscape Power Systems  SourceProductBaseCode=PS
  Terminator : Terminator
  Vrms : Outport
  wires:
  Sequence Analyzer (Phasor)/1 -> Vrms/1
  Vabc/1 -> Sequence Analyzer (Phasor)/1
  Sequence Analyzer (Phasor)/2 -> Terminator/1

== system IEEE33BusTestSystem_DG_Ident/Measurements/Phasor RMS16 ==
  Vabc : Inport
  Sequence Analyzer (Phasor) : powerlib_meascontrol/Measurements/Sequence Analyzer (Phasor)  seq=Positive
      settings: SourceProductName=Simscape Power Systems  SourceProductBaseCode=PS
  Terminator : Terminator
  Vrms : Outport
  wires:
  Sequence Analyzer (Phasor)/1 -> Vrms/1
  Vabc/1 -> Sequence Analyzer (Phasor)/1
  Sequence Analyzer (Phasor)/2 -> Terminator/1

== system IEEE33BusTestSystem_DG_Ident/Measurements/Phasor RMS17 ==
  Vabc : Inport
  Sequence Analyzer (Phasor) : powerlib_meascontrol/Measurements/Sequence Analyzer (Phasor)  seq=Positive
      settings: SourceProductName=Simscape Power Systems  SourceProductBaseCode=PS
  Terminator : Terminator
  Vrms : Outport
  wires:
  Sequence Analyzer (Phasor)/1 -> Vrms/1
  Vabc/1 -> Sequence Analyzer (Phasor)/1
  Sequence Analyzer (Phasor)/2 -> Terminator/1

== system IEEE33BusTestSystem_DG_Ident/Measurements/Phasor RMS18 ==
  Vabc : Inport
  Sequence Analyzer (Phasor) : powerlib_meascontrol/Measurements/Sequence Analyzer (Phasor)  seq=Positive
      settings: SourceProductName=Simscape Power Systems  SourceProductBaseCode=PS
  Terminator : Terminator
  Vrms : Outport
  wires:
  Sequence Analyzer (Phasor)/1 -> Vrms/1
  Vabc/1 -> Sequence Analyzer (Phasor)/1
  Sequence Analyzer (Phasor)/2 -> Terminator/1

== system IEEE33BusTestSystem_DG_Ident/Measurements/Phasor RMS19 ==
  Vabc : Inport
  Sequence Analyzer (Phasor) : powerlib_meascontrol/Measurements/Sequence Analyzer (Phasor)  seq=Positive
      settings: SourceProductName=Simscape Power Systems  SourceProductBaseCode=PS
  Terminator : Terminator
  Vrms : Outport
  wires:
  Sequence Analyzer (Phasor)/1 -> Vrms/1
  Vabc/1 -> Sequence Analyzer (Phasor)/1
  Sequence Analyzer (Phasor)/2 -> Terminator/1

== system IEEE33BusTestSystem_DG_Ident/Measurements/Phasor RMS2 ==
  Vabc : Inport
  Sequence Analyzer (Phasor) : powerlib_meascontrol/Measurements/Sequence Analyzer (Phasor)  seq=Positive
      settings: SourceProductName=Simscape Power Systems  SourceProductBaseCode=PS
  Terminator : Terminator
  Vrms : Outport
  wires:
  Sequence Analyzer (Phasor)/1 -> Vrms/1
  Vabc/1 -> Sequence Analyzer (Phasor)/1
  Sequence Analyzer (Phasor)/2 -> Terminator/1

== system IEEE33BusTestSystem_DG_Ident/Measurements/Phasor RMS20 ==
  Vabc : Inport
  Sequence Analyzer (Phasor) : powerlib_meascontrol/Measurements/Sequence Analyzer (Phasor)  seq=Positive
      settings: SourceProductName=Simscape Power Systems  SourceProductBaseCode=PS
  Terminator : Terminator
  Vrms : Outport
  wires:
  Sequence Analyzer (Phasor)/1 -> Vrms/1
  Vabc/1 -> Sequence Analyzer (Phasor)/1
  Sequence Analyzer (Phasor)/2 -> Terminator/1

== system IEEE33BusTestSystem_DG_Ident/Measurements/Phasor RMS21 ==
  Vabc : Inport
  Sequence Analyzer (Phasor) : powerlib_meascontrol/Measurements/Sequence Analyzer (Phasor)  seq=Positive
      settings: SourceProductName=Simscape Power Systems  SourceProductBaseCode=PS
  Terminator : Terminator
  Vrms : Outport
  wires:
  Sequence Analyzer (Phasor)/1 -> Vrms/1
  Vabc/1 -> Sequence Analyzer (Phasor)/1
  Sequence Analyzer (Phasor)/2 -> Terminator/1

== system IEEE33BusTestSystem_DG_Ident/Measurements/Phasor RMS22 ==
  Vabc : Inport
  Sequence Analyzer (Phasor) : powerlib_meascontrol/Measurements/Sequence Analyzer (Phasor)  seq=Positive
      settings: SourceProductName=Simscape Power Systems  SourceProductBaseCode=PS
  Terminator : Terminator
  Vrms : Outport
  wires:
  Sequence Analyzer (Phasor)/1 -> Vrms/1
  Vabc/1 -> Sequence Analyzer (Phasor)/1
  Sequence Analyzer (Phasor)/2 -> Terminator/1

== system IEEE33BusTestSystem_DG_Ident/Measurements/Phasor RMS23 ==
  Vabc : Inport
  Sequence Analyzer (Phasor) : powerlib_meascontrol/Measurements/Sequence Analyzer (Phasor)  seq=Positive
      settings: SourceProductName=Simscape Power Systems  SourceProductBaseCode=PS
  Terminator : Terminator
  Vrms : Outport
  wires:
  Sequence Analyzer (Phasor)/1 -> Vrms/1
  Vabc/1 -> Sequence Analyzer (Phasor)/1
  Sequence Analyzer (Phasor)/2 -> Terminator/1

== system IEEE33BusTestSystem_DG_Ident/Measurements/Phasor RMS24 ==
  Vabc : Inport
  Sequence Analyzer (Phasor) : powerlib_meascontrol/Measurements/Sequence Analyzer (Phasor)  seq=Positive
      settings: SourceProductName=Simscape Power Systems  SourceProductBaseCode=PS
  Terminator : Terminator
  Vrms : Outport
  wires:
  Sequence Analyzer (Phasor)/1 -> Vrms/1
  Vabc/1 -> Sequence Analyzer (Phasor)/1
  Sequence Analyzer (Phasor)/2 -> Terminator/1

== system IEEE33BusTestSystem_DG_Ident/Measurements/Phasor RMS25 ==
  Vabc : Inport
  Sequence Analyzer (Phasor) : powerlib_meascontrol/Measurements/Sequence Analyzer (Phasor)  seq=Positive
      settings: SourceProductName=Simscape Power Systems  SourceProductBaseCode=PS
  Terminator : Terminator
  Vrms : Outport
  wires:
  Sequence Analyzer (Phasor)/1 -> Vrms/1
  Vabc/1 -> Sequence Analyzer (Phasor)/1
  Sequence Analyzer (Phasor)/2 -> Terminator/1

== system IEEE33BusTestSystem_DG_Ident/Measurements/Phasor RMS26 ==
  Vabc : Inport
  Sequence Analyzer (Phasor) : powerlib_meascontrol/Measurements/Sequence Analyzer (Phasor)  seq=Positive
      settings: SourceProductName=Simscape Power Systems  SourceProductBaseCode=PS
  Terminator : Terminator
  Vrms : Outport
  wires:
  Sequence Analyzer (Phasor)/1 -> Vrms/1
  Vabc/1 -> Sequence Analyzer (Phasor)/1
  Sequence Analyzer (Phasor)/2 -> Terminator/1

== system IEEE33BusTestSystem_DG_Ident/Measurements/Phasor RMS27 ==
  Vabc : Inport
  Sequence Analyzer (Phasor) : powerlib_meascontrol/Measurements/Sequence Analyzer (Phasor)  seq=Positive
      settings: SourceProductName=Simscape Power Systems  SourceProductBaseCode=PS
  Terminator : Terminator
  Vrms : Outport
  wires:
  Sequence Analyzer (Phasor)/1 -> Vrms/1
  Vabc/1 -> Sequence Analyzer (Phasor)/1
  Sequence Analyzer (Phasor)/2 -> Terminator/1

== system IEEE33BusTestSystem_DG_Ident/Measurements/Phasor RMS28 ==
  Vabc : Inport
  Sequence Analyzer (Phasor) : powerlib_meascontrol/Measurements/Sequence Analyzer (Phasor)  seq=Positive
      settings: SourceProductName=Simscape Power Systems  SourceProductBaseCode=PS
  Terminator : Terminator
  Vrms : Outport
  wires:
  Sequence Analyzer (Phasor)/1 -> Vrms/1
  Vabc/1 -> Sequence Analyzer (Phasor)/1
  Sequence Analyzer (Phasor)/2 -> Terminator/1

== system IEEE33BusTestSystem_DG_Ident/Measurements/Phasor RMS29 ==
  Vabc : Inport
  Sequence Analyzer (Phasor) : powerlib_meascontrol/Measurements/Sequence Analyzer (Phasor)  seq=Positive
      settings: SourceProductName=Simscape Power Systems  SourceProductBaseCode=PS
  Terminator : Terminator
  Vrms : Outport
  wires:
  Sequence Analyzer (Phasor)/1 -> Vrms/1
  Vabc/1 -> Sequence Analyzer (Phasor)/1
  Sequence Analyzer (Phasor)/2 -> Terminator/1

== system IEEE33BusTestSystem_DG_Ident/Measurements/Phasor RMS3 ==
  Vabc : Inport
  Sequence Analyzer (Phasor) : powerlib_meascontrol/Measurements/Sequence Analyzer (Phasor)  seq=Positive
      settings: SourceProductName=Simscape Power Systems  SourceProductBaseCode=PS
  Terminator : Terminator
  Vrms : Outport
  wires:
  Sequence Analyzer (Phasor)/1 -> Vrms/1
  Vabc/1 -> Sequence Analyzer (Phasor)/1
  Sequence Analyzer (Phasor)/2 -> Terminator/1

== system IEEE33BusTestSystem_DG_Ident/Measurements/Phasor RMS30 ==
  Vabc : Inport
  Sequence Analyzer (Phasor) : powerlib_meascontrol/Measurements/Sequence Analyzer (Phasor)  seq=Positive
      settings: SourceProductName=Simscape Power Systems  SourceProductBaseCode=PS
  Terminator : Terminator
  Vrms : Outport
  wires:
  Sequence Analyzer (Phasor)/1 -> Vrms/1
  Vabc/1 -> Sequence Analyzer (Phasor)/1
  Sequence Analyzer (Phasor)/2 -> Terminator/1

== system IEEE33BusTestSystem_DG_Ident/Measurements/Phasor RMS31 ==
  Vabc : Inport
  Sequence Analyzer (Phasor) : powerlib_meascontrol/Measurements/Sequence Analyzer (Phasor)  seq=Positive
      settings: SourceProductName=Simscape Power Systems  SourceProductBaseCode=PS
  Terminator : Terminator
  Vrms : Outport
  wires:
  Sequence Analyzer (Phasor)/1 -> Vrms/1
  Vabc/1 -> Sequence Analyzer (Phasor)/1
  Sequence Analyzer (Phasor)/2 -> Terminator/1

== system IEEE33BusTestSystem_DG_Ident/Measurements/Phasor RMS32 ==
  Vabc : Inport
  Sequence Analyzer (Phasor) : powerlib_meascontrol/Measurements/Sequence Analyzer (Phasor)  seq=Positive
      settings: SourceProductName=Simscape Power Systems  SourceProductBaseCode=PS
  Terminator : Terminator
  Vrms : Outport
  wires:
  Sequence Analyzer (Phasor)/1 -> Vrms/1
  Vabc/1 -> Sequence Analyzer (Phasor)/1
  Sequence Analyzer (Phasor)/2 -> Terminator/1

== system IEEE33BusTestSystem_DG_Ident/Measurements/Phasor RMS4 ==
  Vabc : Inport
  Sequence Analyzer (Phasor) : powerlib_meascontrol/Measurements/Sequence Analyzer (Phasor)  seq=Positive
      settings: SourceProductName=Simscape Power Systems  SourceProductBaseCode=PS
  Terminator : Terminator
  Vrms : Outport
  wires:
  Sequence Analyzer (Phasor)/1 -> Vrms/1
  Vabc/1 -> Sequence Analyzer (Phasor)/1
  Sequence Analyzer (Phasor)/2 -> Terminator/1

== system IEEE33BusTestSystem_DG_Ident/Measurements/Phasor RMS5 ==
  Vabc : Inport
  Sequence Analyzer (Phasor) : powerlib_meascontrol/Measurements/Sequence Analyzer (Phasor)  seq=Positive
      settings: SourceProductName=Simscape Power Systems  SourceProductBaseCode=PS
  Terminator : Terminator
  Vrms : Outport
  wires:
  Sequence Analyzer (Phasor)/1 -> Vrms/1
  Vabc/1 -> Sequence Analyzer (Phasor)/1
  Sequence Analyzer (Phasor)/2 -> Terminator/1

== system IEEE33BusTestSystem_DG_Ident/Measurements/Phasor RMS6 ==
  Vabc : Inport
  Sequence Analyzer (Phasor) : powerlib_meascontrol/Measurements/Sequence Analyzer (Phasor)  seq=Positive
      settings: SourceProductName=Simscape Power Systems  SourceProductBaseCode=PS
  Terminator : Terminator
  Vrms : Outport
  wires:
  Sequence Analyzer (Phasor)/1 -> Vrms/1
  Vabc/1 -> Sequence Analyzer (Phasor)/1
  Sequence Analyzer (Phasor)/2 -> Terminator/1

== system IEEE33BusTestSystem_DG_Ident/Measurements/Phasor RMS7 ==
  Vabc : Inport
  Sequence Analyzer (Phasor) : powerlib_meascontrol/Measurements/Sequence Analyzer (Phasor)  seq=Positive
      settings: SourceProductName=Simscape Power Systems  SourceProductBaseCode=PS
  Terminator : Terminator
  Vrms : Outport
  wires:
  Sequence Analyzer (Phasor)/1 -> Vrms/1
  Vabc/1 -> Sequence Analyzer (Phasor)/1
  Sequence Analyzer (Phasor)/2 -> Terminator/1

== system IEEE33BusTestSystem_DG_Ident/Measurements/Phasor RMS8 ==
  Vabc : Inport
  Sequence Analyzer (Phasor) : powerlib_meascontrol/Measurements/Sequence Analyzer (Phasor)  seq=Positive
      settings: SourceProductName=Simscape Power Systems  SourceProductBaseCode=PS
  Terminator : Terminator
  Vrms : Outport
  wires:
  Sequence Analyzer (Phasor)/1 -> Vrms/1
  Vabc/1 -> Sequence Analyzer (Phasor)/1
  Sequence Analyzer (Phasor)/2 -> Terminator/1

== system IEEE33BusTestSystem_DG_Ident/Measurements/Phasor RMS9 ==
  Vabc : Inport
  Sequence Analyzer (Phasor) : powerlib_meascontrol/Measurements/Sequence Analyzer (Phasor)  seq=Positive
      settings: SourceProductName=Simscape Power Systems  SourceProductBaseCode=PS
  Terminator : Terminator
  Vrms : Outport
  wires:
  Sequence Analyzer (Phasor)/1 -> Vrms/1
  Vabc/1 -> Sequence Analyzer (Phasor)/1
  Sequence Analyzer (Phasor)/2 -> Terminator/1
